simulink model "bamquydao"  (R2019a)
settings: Solver=VariableStepAuto  StartTime=0.0  StopTime=3  RelTol=1e-3
settings Model: Creator=dell  LastModifiedBy=dell

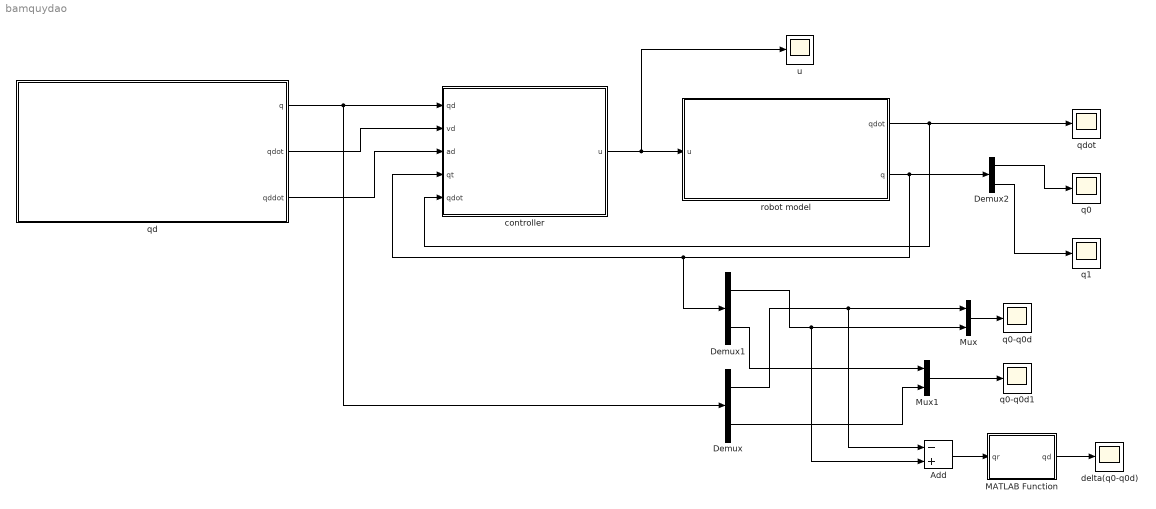
== system bamquydao ==
  Add : Sum  Inputs=-+
  Demux : Demux  Outputs=2
  Demux1 : Demux  Outputs=2
  Demux2 : Demux  Outputs=2
  MATLAB Function : MATLAB Function  TreatAsAtomicUnit=on
  Mux : Mux  Inputs=2
  Mux1 : Mux  Inputs=2
  controller : Subsystem
  delta(q0-q0d) : Scope
  "q0 " : Scope
  q0-q0d : Scope
  q0-q0d1 : Scope
  q1 : Scope
  qd : Subsystem
  qdot : Scope
  robot model : Subsystem
  "u " : Scope
  wires:
  qd/1(q) -> Demux/1, controller/1(qd)
  robot model/2("q ") -> Demux2/1, Demux1/1, controller/4(qt)
  robot model/1(qdot) -> controller/5(qdot), qdot/1
  qd/2(qdot) -> controller/2(vd)
  qd/3(qddot) -> controller/3(ad)
  Demux/1 -> Add/1, Mux/1
  Demux1/1 -> Add/2, Mux/2
  Mux/1 -> q0-q0d/1
  Demux2/1 -> "q0 "/1
  Demux2/2 -> q1/1
  Add/1 -> MATLAB Function/1(qr)
  MATLAB Function/1(qd) -> delta(q0-q0d)/1
  controller/1("u ") -> "u "/1, robot model/1(u)
  Demux1/2 -> Mux1/1
  Demux/2 -> Mux1/2
  Mux1/1 -> q0-q0d1/1

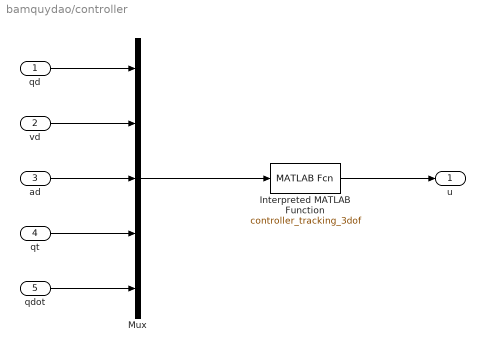
== system bamquydao/controller ==
  qd : Inport
  vd : Inport  Port=2
  ad : Inport  Port=3
  qt : Inport  Port=4
  qdot : Inport  Port=5
  Interpreted MATLAB Function : MATLABFcn  MATLABFcn=controller_tracking_3dof
  Mux : Mux  Inputs=5
  "u " : Outport
  wires:
  Mux/1 -> Interpreted MATLAB Function/1
  qd/1 -> Mux/1
  Interpreted MATLAB Function/1 -> "u "/1
  vd/1 -> Mux/2
  ad/1 -> Mux/3
  qt/1 -> Mux/4
  qdot/1 -> Mux/5

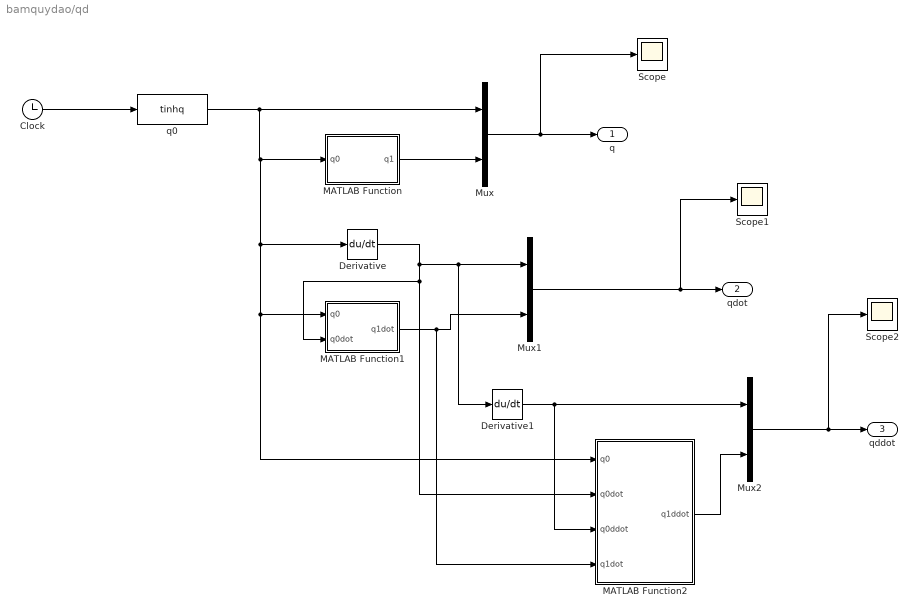
== system bamquydao/qd ==
  Clock : Clock
      settings: Decimation=3
  Derivative : Derivative
  Derivative1 : Derivative
  MATLAB Function : MATLAB Function  TreatAsAtomicUnit=on
  MATLAB Function1 : MATLAB Function  TreatAsAtomicUnit=on
  MATLAB Function2 : MATLAB Function  TreatAsAtomicUnit=on
  Mux : Mux  Inputs=2
  Mux1 : Mux  Inputs=2
  Mux2 : Mux  Inputs=2
  Scope : Scope
  Scope1 : Scope
  Scope2 : Scope
  q0 : MATLABFcn  MATLABFcn=tinhq
  q : Outport
  qdot : Outport  Port=2
  qddot : Outport  Port=3
  wires:
  Clock/1 -> q0/1
  MATLAB Function/1(q1) -> Mux/2
  q0/1 -> MATLAB Function2/1(q0), MATLAB Function1/1(q0), Derivative/1, MATLAB Function/1(q0), Mux/1
  Derivative/1 -> MATLAB Function2/2(q0dot), MATLAB Function1/2(q0dot), Derivative1/1, Mux1/1
  MATLAB Function1/1(q1dot) -> MATLAB Function2/4(q1dot), Mux1/2
  Mux1/1 -> Scope1/1, qdot/1
  Derivative1/1 -> MATLAB Function2/3(q0ddot), Mux2/1
  Mux2/1 -> Scope2/1, qddot/1
  MATLAB Function2/1(q1ddot) -> Mux2/2
  Mux/1 -> q/1, Scope/1

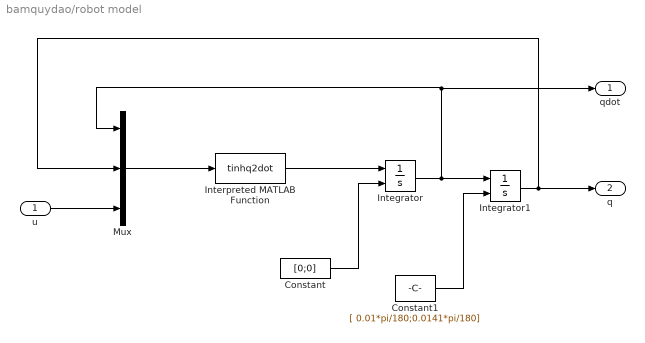
== system bamquydao/robot model ==
  u : Inport
  Constant : Constant  Value=[0;0]
  Constant1 : Constant  Value=[ 0.01*pi/180;0.0141*pi/180]
  Integrator : Integrator  InitialConditionSource=external
  Integrator1 : Integrator  InitialConditionSource=external
  Interpreted MATLAB Function : MATLABFcn  MATLABFcn=tinhq2dot
  Mux : Mux  Inputs=3
  qdot : Outport
  "q " : Outport  Port=2
  wires:
  Mux/1 -> Interpreted MATLAB Function/1
  Integrator/1 -> Mux/1, qdot/1, Integrator1/1
  u/1 -> Mux/3
  Integrator1/1 -> Mux/2, "q "/1
  Interpreted MATLAB Function/1 -> Integrator/1
  Constant/1 -> Integrator/2
  Constant1/1 -> Integrator1/2

== matlab function bamquydao/qd/MATLAB Function1 ==
  data: q0 input; q1dot output; q0dot input
function q1dot = fcn(q0,q0dot)
q1dot=(2*q0dot*(tan(q0^2+1)))/(sqrt(2)*tan(q0^2+1));

== matlab function bamquydao/qd/MATLAB Function ==
  data: q0 input; q1 output
function q1 = fcn(q0)
q1=2*atan((1/sqrt(2))*tan(q0));

== matlab function bamquydao/qd/MATLAB Function2 ==
  data: q0 input; q1ddot output; q0dot input; q0ddot input; q1dot input
function q1ddot = fcn(q0,q0dot,q0ddot,q1dot)
q1ddot=((2*tan(q0)^2+1)*(q0ddot+2*q0dot^2*tan(q0))-0.5*q1dot^2*tan(q0)*(tan(q0)^2+2))/(sqrt(2)*(tan(q0)^2+2));
% q1ddot=(2^(1/2)*(q0ddot*(tan(q0)^2 + 1) + 2*q0dot*tan(q0)*(tan(q0)^2 + 1) - 2^(1/2)*q1dot*tan(q1/2)*(tan(q1/2)^2/2 + 1/2)))/(tan(q1/2)^2 + 1);

== matlab function bamquydao/MATLAB Function ==
  data: qr input; qd output
function qd = fcn(qr)
qd=qr*180/pi;
